simulink model "PWMGenerator"  (R2020a)
settings: Solver=FixedStepAuto  StartTime=0.0  StopTime=0.05  FixedStep=2e-08  RelTol=1e-3
undefined symbols (not defined in the file): Down, Fsw, GateVoltage, PWMResolution, Up
libraries: eeGeneralControl x1
settings Model: Creator=ykamatan  LastModifiedBy=ykamatan
settings SolverCC: MaxConsecutiveMinStep=10
settings DataIOCC: SaveOutput=off  SaveTime=off

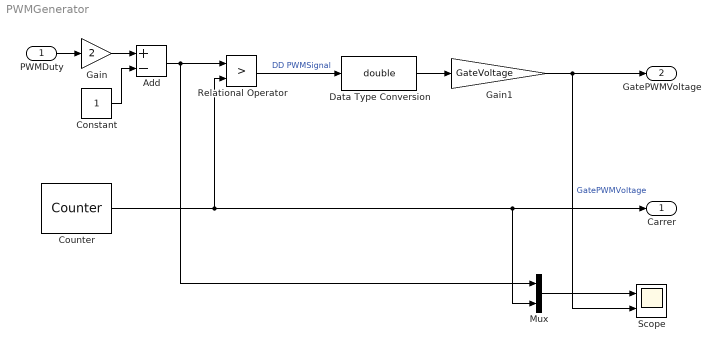
== system PWMGenerator ==
  PWMDuty : Inport  OutDataTypeStr=double  PortDimensions=1
  Add : Sum  Inputs=+-
  Constant : Constant
  Counter : eeGeneralControl/Counter  CarrCount=Up-Down  Range=[-1 1]  Tper=1/Fsw/2  Tdelay=0  Ts=1/Fsw*PWMResolution
      settings: SourceProductBaseCode=PS
  Data Type Conversion : DataTypeConversion  OutDataTypeStr=double
  Gain : Gain  Gain=2
  Gain1 : Gain  Gain=GateVoltage
  Mux : Mux  Inputs=2
  Relational Operator : RelationalOperator  Operator=>  OutDataTypeStr=boolean  RndMeth=Simplest
  Scope : Scope  NumInputPorts=2
  Carrer : Outport  OutDataTypeStr=double  PortDimensions=1  SampleTime=[2e-08,0]
  GatePWMVoltage : Outport  Port=2  OutDataTypeStr=double  PortDimensions=1  SampleTime=[2e-08,0]
  wires:
  Add/1 -> Mux/1, Relational Operator/1
  Constant/1 -> Add/2
  Counter/1 -> Relational Operator/2, Mux/2, Carrer/1
  PWMDuty/1 -> Gain/1
  Gain/1 -> Add/1
  Relational Operator/1 -> Data Type Conversion/1  "DD PWMSignal"
  Data Type Conversion/1 -> Gain1/1
  Gain1/1 -> Scope/2, GatePWMVoltage/1  "GatePWMVoltage"
  Mux/1 -> Scope/1
